simulink library "SimFly_Motors"  (R2015b)
settings: Solver=VariableStepAuto  StartTime=0.0  StopTime=10.0  RelTol=1e-3
settings Model: Creator=mocherma  LastModifiedBy=marcell

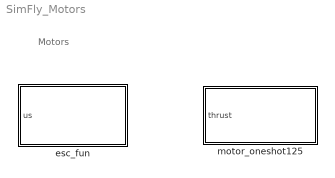
== system SimFly_Motors ==
  note: Motors
  esc_fun : MATLAB Function  TreatAsAtomicUnit=on  mask(SimFly ESC){esc_num=4, esc_sample_time=-1}
      mask prompts: esc_num "Number of ESC"; esc_sample_time "Sample Time"
      mask help: Writes microseconds values to ESCs
  motor_oneshot125 : MATLAB Function  TreatAsAtomicUnit=on  mask(SImFly){Pin_number=1, oneshot_sample=1/500}
      mask prompts: Pin_number "Pin number for motor output (1-8)"; oneshot_sample "Sample Time"
      mask help:
      | Block for Motor output with oneshot signal
      |
      | Input = value between 0 - 1 [0 - 100% thrust]
      | 0 = 125 Microseconds PWM
      | 1 = 250 Microseconds PWM

== matlab function SimFly_Motors/motor_oneshot125 ==
  settings: updateMethod=DISCRETE  sampleTime=oneshot_sample
  data: thrust input; Pin_number parameter
function oneshot_send(thrust, Pin_number)
%PURPOSE: Sends a pwm signal to specified pin
%AUTHOR: Marcell Mocher
%DATE: 10.6.2016
%VERSION: 0.1 V Fist build
%Input: - thrust[x,1] = percent to esc
%Info: This drive requires function call triggered simuluink functions in
% order to work
%Requires:  _servo_attach
%           _servo_write_us


persistent init_flag

% Mask parameters

esc_num = uint8(Pin_number);

if strcmp(coder.target,'rtw')
    if isempty(init_flag)
    init_flag = true;   
    coder.ceval('oneshot125_init',esc_num);    
    end
    pwm_leght = 130 * thrust + 120;
    coder.ceval('oneshot125',esc_num,uint8(pwm_leght));
end

== matlab function SimFly_Motors/esc_fun ==
  settings: updateMethod=DISCRETE  sampleTime=esc_sample_time
  data: us input; esc_num parameter
function esc_write_us(us, esc_num)
%PURPOSE: Reads PWM signals from receiver
%AUTHOR: Marcell Mocher
%DATE: 10.6.2016
%VERSION: 0.1 V Fist build
%Input: - us[x,1] = microseconds to esc
%Info: This drive requires function call triggered simuluink functions in
% order to work
%Requires:  _servo_attach
%           _servo_write_us

persistent init_flag

% Mask parameters

esc_num = uint8(esc_num);

if strcmp(coder.target,'rtw')
    if isempty(init_flag)
        init_flag = 1;
        for i = 1:esc_num
        coder.ceval('_servo_attach',uint8(i));
        end
    end
    
    for i = 1:esc_num
    coder.ceval('_servo_write_us',uint8(i),uint32(us(i)));
    end
    
else
    
    
end
